simulink model "power_controller_test_simu"  (R2023b)
settings: Solver=VariableStepAuto  StartTime=0.0  StopTime=30  RelTol=1e-3
undefined symbols (not defined in the file): cp_max, lambda_opt, omega_WTR_min, omega_WTR_n, omega_WTR_sl, R_WTR
settings Model: Creator=Martin Pedersen  LastModifiedBy=Martin Pedersen

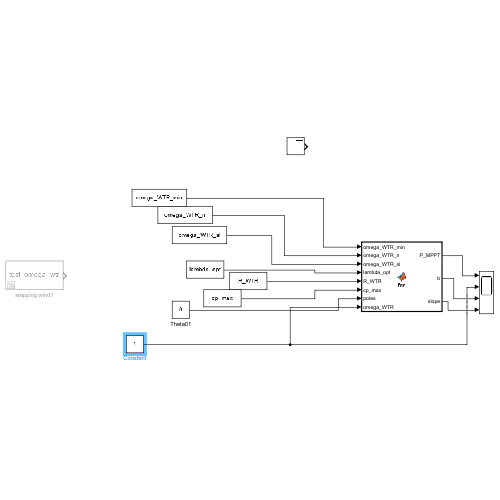
[thumbnail: Simulink's stored preview of the top-level diagram]
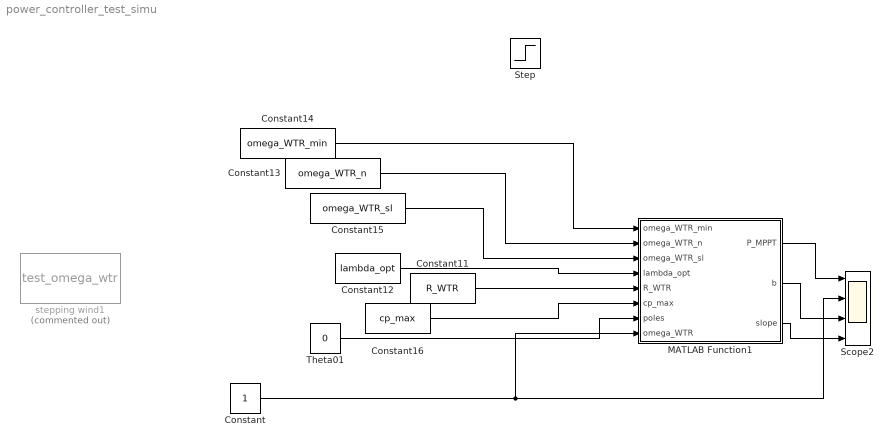
== system power_controller_test_simu ==
  Constant : Constant
  Constant11 : Constant  Value=R_WTR
  Constant12 : Constant  Value=lambda_opt
  Constant13 : Constant  Value=omega_WTR_n
  Constant14 : Constant  Value=omega_WTR_min
  Constant15 : Constant  Value=omega_WTR_sl
  Constant16 : Constant  Value=cp_max
  MATLAB Function1 : MATLAB Function  TreatAsAtomicUnit=on
  Scope2 : Scope  NumInputPorts=4
  Step : Step  Time=5  Before=0.6  SampleTime=0
  Theta01 : Constant  Value=0
  stepping wind1 : FromWorkspace  Commented=on  VariableName=test_omega_wtr  OutputAfterFinalValue=Holding final value
  wires:
  Constant12/1 -> MATLAB Function1/4(lambda_opt)
  Constant11/1 -> MATLAB Function1/5(R_WTR)
  Theta01/1 -> MATLAB Function1/7(poles)
  MATLAB Function1/1(P_MPPT) -> Scope2/1
  Constant15/1 -> MATLAB Function1/3(omega_WTR_sl)
  Constant16/1 -> MATLAB Function1/6(cp_max)
  Constant14/1 -> MATLAB Function1/1(omega_WTR_min)
  Constant13/1 -> MATLAB Function1/2(omega_WTR_n)
  Constant/1 -> Scope2/2, MATLAB Function1/8(omega_WTR)
  MATLAB Function1/2(b) -> Scope2/3
  MATLAB Function1/3(slope) -> Scope2/4

== matlab function power_controller_test_simu/MATLAB Function1 ==
  data: omega_WTR_min input; P_MPPT output; omega_WTR_n input; omega_WTR_sl input; lambda_opt input; R_WTR input; cp_max input; poles input; omega_WTR input; b output; slope output
function [P_MPPT,b,slope] = fcn(omega_WTR_min,omega_WTR_n,omega_WTR_sl,lambda_opt,R_WTR,cp_max,poles,omega_WTR)

rho = 1.2225;
P_mppt_sl = 0.5*pi*rho*R_WTR^5*cp_max/lambda_opt^3*omega_WTR_sl^3; %
P_mppt_max = 0.5*pi*rho*R_WTR^5*cp_max/lambda_opt^3*omega_WTR_n^3;
slope = (P_mppt_max-P_mppt_sl)/(omega_WTR_n-omega_WTR_sl);
b = P_mppt_max-slope*omega_WTR_n;

if omega_WTR < omega_WTR_min
    y = 0;
elseif omega_WTR < omega_WTR_sl
    y = 0.5*pi*rho*R_WTR^5*cp_max/lambda_opt^3*omega_WTR^3;
elseif omega_WTR < omega_WTR_n
    y = slope*omega_WTR+b;
else
    y = 0.5*pi*rho*R_WTR^5*cp_max/lambda_opt^3*omega_WTR_n^3;

end

P_MPPT = y ;
